simulink model "ex_bus_to_vector"  (Simulink 10.0)
settings: Solver=ode3  StartTime=0.0  StopTime=10.0  FixedStep=1  MaxStep=1  RelTol=1e-3  EnableMultiTasking=on
libraries: simulink x1
settings Model: Creator=The MathWorks, Inc.  LastModifiedBy=bhisma
settings DataIOCC: LimitDataPoints=on
settings OptimizationCC: ExpressionDepthLimit=2147483647
settings DebuggingCC: FcnCallInpInsideContextMsg=warning  StateNameClashWarn=warning
settings GRTTargetCC: GeneratePreprocessorConditionals=Disable all  CombineOutputUpdateFcns=on  GRTInterface=off
settings ConfigComp: CovExternalEMLEnable=off

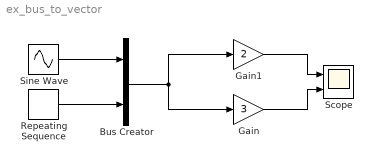
== system ex_bus_to_vector ==
  Bus Creator : BusCreator  Inputs=2
  Gain : Gain  Gain=3
  Gain1 : Gain  Gain=2
  Repeating Sequence : simulink/Sources/Repeating Sequence  rep_seq_t=[0 2]  rep_seq_y=[0 2]
  Scope : Scope  NumInputPorts=2
  Sine Wave : Sin  SampleTime=0
  wires:
  Repeating Sequence/1 -> Bus Creator/2
  Gain1/1 -> Scope/1
  Sine Wave/1 -> Bus Creator/1
  Bus Creator/1 -> Gain/1, Gain1/1
  Gain/1 -> Scope/2
